simulink model "ArrayMaker"  (R2021a)
settings: Solver=FixedStepAuto  StartTime=0.0  StopTime=inf  RelTol=1e-3
model workspace (MAT data in the model file):
  Logfile_Data_Object = robotics.ros.BagSelection
  Logfile_Data_Object.FilePath = 'C:\Users\yekat\Documents\MATLAB source files\Pioneer Files\Rosbag files\November\01.11.22\Point A-B part 1.bag'
  Logfile_Data_Object.StartTime = 1663346854.77
  Logfile_Data_Object.EndTime = 1663347023.11
  Logfile_Data_Object.NumMessages = 14261
  Logfile_Data_Object.AvailableTopics = table
  Logfile_Data_Object.AvailableTopics.data{1} = [1; 1681; 1681; 1385; 1; 1; 1; 1682; 1681; 1682; 1397; 1385; 1683]
  Logfile_Data_Object.AvailableTopics.data{2} = categorical
  Logfile_Data_Object.AvailableTopics.data{2}.categoryNames = {'dynamic_reconfigure/Config'; 'dynamic_reconfigure/ConfigDescription'; 'geometry_msgs/Twist'; 'nav_msgs/Odometry'; 'rosaria/BumperState'; 'rosgraph_msgs/Log'; 'sensor_msgs/PointCloud'; 'sensor_msgs/PointCloud2'; 'std_msgs/Bool'; 'std_msgs/Float64'; 'std_msgs/Int8'; 'tf2_msgs/TFMessage'}
  Logfile_Data_Object.AvailableTopics.data{2}.codes = [11; 10; 5; 3; 9; 2; 1; 4; 7; 8; 6; 6; 12]
  Logfile_Data_Object.AvailableTopics.data{3}{1} = ''
  Logfile_Data_Object.AvailableTopics.data{3}{2} = ''
  Logfile_Data_Object.AvailableTopics.data{3}{3} = '  uint32 Seq
    |   Time Stamp
    |   char FrameId
    | logical[] FrontBumpers
    | logical[] RearBumpers
    | '
  Logfile_Data_Object.AvailableTopics.data{3}{4} = '  double X
    |   double Y
    |   double Z
    | geometry_msgs/Vector3 Angular
    |   double X
    |   double Y
    |   double Z
    | '
  Logfile_Data_Object.AvailableTopics.data{3}{5} = ''
  Logfile_Data_Object.AvailableTopics.data{3}{6} = '  char Name
    |   char Type
    |   dynamic_reconfigure/ParamDescription[] Parameters
    |     char Name
    |     char Type
    |     uint32 Level
    |     char Description
    |     char EditMethod
    |   int32 Parent
    |   int32 Id
    | dynamic_reconfigure/Config Max
    |   dynamic_reconfigure/BoolParameter[] Bools
    |     char Name
    |     logical Value
    |   dynamic_reconfigure/IntParameter[] Ints
    |     char Name
    |     int32 Value
    |   dynamic_reconfigure/StrParameter[] Strs
    |     char Name
    |     char Value
    |   dynamic_reconfigure/DoubleParameter[] Doubles
    |     char Name
    |     double Value
    |   dynamic_reconfigure/GroupState[] Groups
    |     char Name
    |     logical State
    |     int32 Id
    |     int32 Parent
    | dynamic_reconfigure/Config Min
    |   dynamic_reconfigure/BoolParameter[] Bools
    |     char Name
    |     logical Value
    |   dynamic_reconfigure/IntParameter[] Ints
    |     char Name
    |     int32 Value
    |   dynamic_reconfigure/StrParameter[] Strs
    |     char Name
    |     char Value
    |   dynamic_reconfigure/DoubleParameter[] Doubles
    |     char Name
    |     double Value
    |   dynamic_reconfigure/GroupState[] Groups
    |     char Name
    |     logical State
    |     int32 Id
    |     int32 Parent
    | dynamic_reconfigure/Config Dflt
    |   dynamic_reconfigure/BoolParameter[] Bools
    |     char Name
    |     logical Value
    |   dynamic_reconfigure/IntParameter[] Ints
    |     char Name
    |     int32 Value
    |   dynamic_reconfigure/StrParameter[] Strs
    |     char Name
    |     char Value
    |   dynamic_reconfigure/DoubleParameter[] Doubles
    |     char Name
    |     double Value
    |   dynamic_reconfigure/GroupState[] Groups
    |     char Name
    |     logical State
    |     int32 Id
    |     int32 Parent
    | '
  Logfile_Data_Object.AvailableTopics.data{3}{7} = '  char Name
    |   logical Value
    | dynamic_reconfigure/IntParameter[] Ints
    |   char Name
    |   int32 Value
    | dynamic_reconfigure/StrParameter[] Strs
    |   char Name
    |   char Value
    | dynamic_reconfigure/DoubleParameter[] Doubles
    |   char Name
    |   double Value
    | dynamic_reconfigure/GroupState[] Groups
    |   char Name
    |   logical State
    |   int32 Id
    |   int32 Parent
    | '
  Logfile_Data_Object.AvailableTopics.data{3}{8} = '  uint32 Seq
    |   Time Stamp
    |   char FrameId
    | char ChildFrameId
    | geometry_msgs/PoseWithCovariance Pose
    |   geometry_msgs/Pose Pose
    |     geometry_msgs/Point Position
    |       double X
    |       double Y
    |       double Z
    |     geometry_msgs/Quaternion Orientation
    |       double X
    |       double Y
    |       double Z
    |       double W
    |   double[36] Covariance
    | geometry_msgs/TwistWithCovariance Twist
    |   geometry_msgs/Twist Twist
    |     geometry_msgs/Vector3 Linear
    |       double X
    |       double Y
    |       double Z
    |     geometry_msgs/Vector3 Angular
    |       double X
    |       double Y
    |       double Z
    |   double[36] Covariance
    | '
  Logfile_Data_Object.AvailableTopics.data{3}{9} = '  uint32 Seq
    |   Time Stamp
    |   char FrameId
    | geometry_msgs/Point32[] Points
    |   single X
    |   single Y
    |   single Z
    | sensor_msgs/ChannelFloat32[] Channels
    |   char Name
    |   single[] Values
    | '
  Logfile_Data_Object.AvailableTopics.data{3}{10} = '  uint32 Seq
    |   Time Stamp
    |   char FrameId
    | uint32 Height
    | uint32 Width
    | sensor_msgs/PointField[] Fields
    |   uint8 INT8
    |   uint8 UINT8
    |   uint8 INT16
    |   uint8 UINT16
    |   uint8 INT32
    |   uint8 UINT32
    |   uint8 FLOAT32
    |   uint8 FLOAT64
    |   char Name
    |   uint32 Offset
    |   uint8 Datatype
    |   uint32 Count
    | logical IsBigendian
    | uint32 PointStep
    | uint32 RowStep
    | uint8[] Data
    | logical IsDense
    | '
  Logfile_Data_Object.AvailableTopics.data{3}{11} = 'int8 INFO
    | int8 WARN
    | int8 ERROR
    | int8 FATAL
    | std_msgs/Header Header
    |   uint32 Seq
    |   Time Stamp
    |   char FrameId
    | int8 Level
    | char Name
    | char Msg
    | char File
    | char Function
    | uint32 Line
    | char[] Topics
    | '
  Logfile_Data_Object.AvailableTopics.data{3}{12} = 'int8 INFO
    | int8 WARN
    | int8 ERROR
    | int8 FATAL
    | std_msgs/Header Header
    |   uint32 Seq
    |   Time Stamp
    |   char FrameId
    | int8 Level
    | char Name
    | char Msg
    | char File
    | char Function
    | uint32 Line
    | char[] Topics
    | '
  Logfile_Data_Object.AvailableTopics.data{3}{13} = '  std_msgs/Header Header
    |     uint32 Seq
    |     Time Stamp
    |     char FrameId
    |   char ChildFrameId
    |   geometry_msgs/Transform Transform
    |     geometry_msgs/Vector3 Translation
    |       double X
    |       double Y
    |       double Z
    |     geometry_msgs/Quaternion Rotation
    |       double X
    |       double Y
    |       double Z
    |       double W
    | '
  Logfile_Data_Object.AvailableTopics.ndims = 2
  Logfile_Data_Object.AvailableTopics.nrows = 13
  Logfile_Data_Object.AvailableTopics.rownames = {'/RosAria/battery_recharge_state'; '/RosAria/battery_voltage'; '/RosAria/bumper_state'; '/RosAria/cmd_vel'; '/RosAria/motors_state'; '/RosAria/parameter_descriptions'; '/RosAria/parameter_updates'; '/RosAria/pose'; '/RosAria/sonar'; '/RosAria/sonar_pointcloud2'; '/rosout'; '/rosout_agg'; '/tf'}
  Logfile_Data_Object.AvailableTopics.nvars = 3
  Logfile_Data_Object.AvailableTopics.varnames = {'NumMessages', 'MessageType', 'MessageDefinition'}
  Logfile_Data_Object.AvailableTopics.props.useVariableNamesOriginal = 0
  Logfile_Data_Object.AvailableTopics.props.useDimensionNamesOriginal = 0
  Logfile_Data_Object.AvailableTopics.props.CustomProps = struct()
  Logfile_Data_Object.AvailableTopics.props.VariableCustomProps = struct()
  Logfile_Data_Object.AvailableTopics.props.versionSavedFrom = 4
  Logfile_Data_Object.AvailableTopics.props.minCompatibleVersion = 1
  Logfile_Data_Object.AvailableTopics.props.incompatibilityMsg = ''
  Logfile_Data_Object.AvailableTopics.props.VersionSavedFrom = 4
  Logfile_Data_Object.AvailableTopics.props.Description = ''
  Logfile_Data_Object.AvailableTopics.props.VariableNamesOriginal = {}
  Logfile_Data_Object.AvailableTopics.props.DimensionNames = {'Row', 'Variables'}
  Logfile_Data_Object.AvailableTopics.props.DimensionNamesOriginal = {}
  Logfile_Data_Object.AvailableTopics.props.UserData = []
  Logfile_Data_Object.AvailableTopics.props.VariableDescriptions = {}
  Logfile_Data_Object.AvailableTopics.props.VariableUnits = {}
  Logfile_Data_Object.AvailableTopics.props.VariableContinuity = {}
  Logfile_Data_Object.AvailableFrames = {'base_link'; 'odom'}
  Logfile_Data_Object.MessageList = table
  Logfile_Data_Object.MessageList.data{1} = [1663346854.77 1663346854.77 1663346854.77 1663346854.77 1663346854.77 1663346854.77 1663346854.77 1663346854.77 1663346854.77 1663346854.77 1663346854.78 1663346854.78 ... (14261 elements, 14261x1)]
  Logfile_Data_Object.MessageList.data{2} = categorical
  Logfile_Data_Object.MessageList.data{2}.categoryNames = {'/RosAria/battery_recharge_state'; '/RosAria/battery_voltage'; '/RosAria/bumper_state'; '/RosAria/cmd_vel'; '/RosAria/motors_state'; '/RosAria/parameter_descriptions'; '/RosAria/parameter_updates'; '/RosAria/pose'; '/RosAria/sonar'; '/RosAria/sonar_pointcloud2'; '/rosout'; '/rosout_agg'; '/tf'}
  Logfile_Data_Object.MessageList.data{2}.codes = [11 11 11 11 11 11 11 11 11 11 6 5 ... (14261 elements, 14261x1)]
  Logfile_Data_Object.MessageList.data{3} = categorical
  Logfile_Data_Object.MessageList.data{3}.categoryNames = {'std_msgs/Int8'; 'std_msgs/Float64'; 'rosaria/BumperState'; 'geometry_msgs/Twist'; 'std_msgs/Bool'; 'dynamic_reconfigure/ConfigDescription'; 'dynamic_reconfigure/Config'; 'nav_msgs/Odometry'; 'sensor_msgs/PointCloud'; 'sensor_msgs/PointCloud2'; 'rosgraph_msgs/Log'; 'tf2_msgs/TFMessage'}
  Logfile_Data_Object.MessageList.data{3}.codes = [11 11 11 11 11 11 11 11 11 11 6 5 ... (14261 elements, 14261x1)]
  Logfile_Data_Object.MessageList.data{4} = [5486 5746 6002 6281 6566 6840 7104 7381 7665 7932 9864 11694 ... (14261 elements, 14261x1)]
  Logfile_Data_Object.MessageList.ndims = 2
  Logfile_Data_Object.MessageList.nrows = 14261
  Logfile_Data_Object.MessageList.nvars = 4
  Logfile_Data_Object.MessageList.varnames = {'Time', 'Topic', 'MessageType', 'FileOffset'}
  Logfile_Data_Object.MessageList.props.useVariableNamesOriginal = 0
  Logfile_Data_Object.MessageList.props.useDimensionNamesOriginal = 0
  Logfile_Data_Object.MessageList.props.CustomProps = struct()
  Logfile_Data_Object.MessageList.props.VariableCustomProps = struct()
  Logfile_Data_Object.MessageList.props.versionSavedFrom = 4
  Logfile_Data_Object.MessageList.props.minCompatibleVersion = 1
  Logfile_Data_Object.MessageList.props.incompatibilityMsg = ''
  Logfile_Data_Object.MessageList.props.VersionSavedFrom = 4
  Logfile_Data_Object.MessageList.props.Description = ''
  Logfile_Data_Object.MessageList.props.VariableNamesOriginal = {}
  Logfile_Data_Object.MessageList.props.DimensionNames = {'Row', 'Variables'}
  Logfile_Data_Object.MessageList.props.DimensionNamesOriginal = {}
  Logfile_Data_Object.MessageList.props.UserData = []
  Logfile_Data_Object.MessageList.props.VariableDescriptions = {}
  Logfile_Data_Object.MessageList.props.VariableUnits = {}
  Logfile_Data_Object.MessageList.props.VariableContinuity = {}
  Logfile_Data_Object.TopicTypeMap = containers.Map
  Logfile_Data_Object.TopicTypeMap.serialization.keys = {'/RosAria/battery_recharge_state', '/RosAria/battery_voltage', '/RosAria/bumper_state', '/RosAria/cmd_vel', '/RosAria/motors_state', '/RosAria/parameter_descriptions', '/RosAria/parameter_updates', '/RosAria/pose', '/RosAria/sonar', '/RosAria/sonar_pointcloud2', '/rosout', '/rosout_agg', '/tf'}
  Logfile_Data_Object.TopicTypeMap.serialization.values = {'std_msgs/Int8', 'std_msgs/Float64', 'rosaria/BumperState', 'geometry_msgs/Twist', 'std_msgs/Bool', 'dynamic_reconfigure/ConfigDescription', 'dynamic_reconfigure/Config', 'nav_msgs/Odometry', 'sensor_msgs/PointCloud', 'sensor_msgs/PointCloud2', 'rosgraph_msgs/Log', 'rosgraph_msgs/Log', 'tf2_msgs/TFMessage'}
  Logfile_Data_Object.TopicTypeMap.serialization.uniformity = 1
  Logfile_Data_Object.TopicTypeMap.serialization.keyType = 'char'
  Logfile_Data_Object.TopicTypeMap.serialization.valueType = 'char'
  Logfile_Data_Object.TopicDefinitionMap = containers.Map
  Logfile_Data_Object.TopicDefinitionMap.serialization.keys = {'/RosAria/battery_recharge_state', '/RosAria/battery_voltage', '/RosAria/bumper_state', '/RosAria/cmd_vel', '/RosAria/motors_state', '/RosAria/parameter_descriptions', '/RosAria/parameter_updates', '/RosAria/pose', '/RosAria/sonar', '/RosAria/sonar_pointcloud2', '/rosout', '/rosout_agg', '/tf'}
  Logfile_Data_Object.TopicDefinitionMap.serialization.values{1} = ''
  Logfile_Data_Object.TopicDefinitionMap.serialization.values{2} = ''
  Logfile_Data_Object.TopicDefinitionMap.serialization.values{3} = '  uint32 Seq
    |   Time Stamp
    |   char FrameId
    | logical[] FrontBumpers
    | logical[] RearBumpers
    | '
  Logfile_Data_Object.TopicDefinitionMap.serialization.values{4} = '  double X
    |   double Y
    |   double Z
    | geometry_msgs/Vector3 Angular
    |   double X
    |   double Y
    |   double Z
    | '
  Logfile_Data_Object.TopicDefinitionMap.serialization.values{5} = ''
  Logfile_Data_Object.TopicDefinitionMap.serialization.values{6} = '  char Name
    |   char Type
    |   dynamic_reconfigure/ParamDescription[] Parameters
    |     char Name
    |     char Type
    |     uint32 Level
    |     char Description
    |     char EditMethod
    |   int32 Parent
    |   int32 Id
    | dynamic_reconfigure/Config Max
    |   dynamic_reconfigure/BoolParameter[] Bools
    |     char Name
    |     logical Value
    |   dynamic_reconfigure/IntParameter[] Ints
    |     char Name
    |     int32 Value
    |   dynamic_reconfigure/StrParameter[] Strs
    |     char Name
    |     char Value
    |   dynamic_reconfigure/DoubleParameter[] Doubles
    |     char Name
    |     double Value
    |   dynamic_reconfigure/GroupState[] Groups
    |     char Name
    |     logical State
    |     int32 Id
    |     int32 Parent
    | dynamic_reconfigure/Config Min
    |   dynamic_reconfigure/BoolParameter[] Bools
    |     char Name
    |     logical Value
    |   dynamic_reconfigure/IntParameter[] Ints
    |     char Name
    |     int32 Value
    |   dynamic_reconfigure/StrParameter[] Strs
    |     char Name
    |     char Value
    |   dynamic_reconfigure/DoubleParameter[] Doubles
    |     char Name
    |     double Value
    |   dynamic_reconfigure/GroupState[] Groups
    |     char Name
    |     logical State
    |     int32 Id
    |     int32 Parent
    | dynamic_reconfigure/Config Dflt
    |   dynamic_reconfigure/BoolParameter[] Bools
    |     char Name
    |     logical Value
    |   dynamic_reconfigure/IntParameter[] Ints
    |     char Name
    |     int32 Value
    |   dynamic_reconfigure/StrParameter[] Strs
    |     char Name
    |     char Value
    |   dynamic_reconfigure/DoubleParameter[] Doubles
    |     char Name
    |     double Value
    |   dynamic_reconfigure/GroupState[] Groups
    |     char Name
    |     logical State
    |     int32 Id
    |     int32 Parent
    | '
  Logfile_Data_Object.TopicDefinitionMap.serialization.values{7} = '  char Name
    |   logical Value
    | dynamic_reconfigure/IntParameter[] Ints
    |   char Name
    |   int32 Value
    | dynamic_reconfigure/StrParameter[] Strs
    |   char Name
    |   char Value
    | dynamic_reconfigure/DoubleParameter[] Doubles
    |   char Name
    |   double Value
    | dynamic_reconfigure/GroupState[] Groups
    |   char Name
    |   logical State
    |   int32 Id
    |   int32 Parent
    | '
  Logfile_Data_Object.TopicDefinitionMap.serialization.values{8} = '  uint32 Seq
    |   Time Stamp
    |   char FrameId
    | char ChildFrameId
    | geometry_msgs/PoseWithCovariance Pose
    |   geometry_msgs/Pose Pose
    |     geometry_msgs/Point Position
    |       double X
    |       double Y
    |       double Z
    |     geometry_msgs/Quaternion Orientation
    |       double X
    |       double Y
    |       double Z
    |       double W
    |   double[36] Covariance
    | geometry_msgs/TwistWithCovariance Twist
    |   geometry_msgs/Twist Twist
    |     geometry_msgs/Vector3 Linear
    |       double X
    |       double Y
    |       double Z
    |     geometry_msgs/Vector3 Angular
    |       double X
    |       double Y
    |       double Z
    |   double[36] Covariance
    | '
  Logfile_Data_Object.TopicDefinitionMap.serialization.values{9} = '  uint32 Seq
    |   Time Stamp
    |   char FrameId
    | geometry_msgs/Point32[] Points
    |   single X
    |   single Y
    |   single Z
    | sensor_msgs/ChannelFloat32[] Channels
    |   char Name
    |   single[] Values
    | '
  Logfile_Data_Object.TopicDefinitionMap.serialization.values{10} = '  uint32 Seq
    |   Time Stamp
    |   char FrameId
    | uint32 Height
    | uint32 Width
    | sensor_msgs/PointField[] Fields
    |   uint8 INT8
    |   uint8 UINT8
    |   uint8 INT16
    |   uint8 UINT16
    |   uint8 INT32
    |   uint8 UINT32
    |   uint8 FLOAT32
    |   uint8 FLOAT64
    |   char Name
    |   uint32 Offset
    |   uint8 Datatype
    |   uint32 Count
    | logical IsBigendian
    | uint32 PointStep
    | uint32 RowStep
    | uint8[] Data
    | logical IsDense
    | '
  Logfile_Data_Object.TopicDefinitionMap.serialization.values{11} = 'int8 INFO
    | int8 WARN
    | int8 ERROR
    | int8 FATAL
    | std_msgs/Header Header
    |   uint32 Seq
    |   Time Stamp
    |   char FrameId
    | int8 Level
    | char Name
    | char Msg
    | char File
    | char Function
    | uint32 Line
    | char[] Topics
    | '
  Logfile_Data_Object.TopicDefinitionMap.serialization.values{12} = 'int8 INFO
    | int8 WARN
    | int8 ERROR
    | int8 FATAL
    | std_msgs/Header Header
    |   uint32 Seq
    |   Time Stamp
    |   char FrameId
    | int8 Level
    | char Name
    | char Msg
    | char File
    | char Function
    | uint32 Line
    | char[] Topics
    | '
  Logfile_Data_Object.TopicDefinitionMap.serialization.values{13} = '  std_msgs/Header Header
    |     uint32 Seq
    |     Time Stamp
    |     char FrameId
    |   char ChildFrameId
    |   geometry_msgs/Transform Transform
    |     geometry_msgs/Vector3 Translation
    |       double X
    |       double Y
    |       double Z
    |     geometry_msgs/Quaternion Rotation
    |       double X
    |       double Y
    |       double Z
    |       double W
    | '
  Logfile_Data_Object.TopicDefinitionMap.serialization.uniformity = 1
  Logfile_Data_Object.TopicDefinitionMap.serialization.keyType = 'char'
  Logfile_Data_Object.TopicDefinitionMap.serialization.valueType = 'char'
  Logfile_Data_Object.messageTypeMap = containers.Map
  Logfile_Data_Object.messageTypeMap.serialization.keys = {}
  Logfile_Data_Object.messageTypeMap.serialization.values = {}
  Logfile_Data_Object.messageTypeMap.serialization.uniformity = 0
  Logfile_Data_Object.messageTypeMap.serialization.keyType = 'char'
  Logfile_Data_Object.messageTypeMap.serialization.valueType = 'any'
  Logfile_Data_Object.Parser = robotics.ros.internal.tf.TransformationTreeParser
  Logfile_Data_Object.Parser.UseObjectMsg = 1
  Logfile_Path = 'C:\Users\yekat\Documents\MATLAB source files\Pioneer Files\Rosbag files\November\01.11.22\Point A-B part 1.bag'
  Logfile_Playback_Duration = nan
  Logfile_Playback_Offset = nan
libraries: robotlib x2
settings Model: Creator=yekat  LastModifiedBy=yekat
settings OptimizationCC: EnhancedBackFolding=on  PassReuseOutputArgsAs=Individual arguments  ZeroExternalMemoryAtStartup=off  ZeroInternalMemoryAtStartup=off  MaxStackSize=64  OptimizeBlockOrder=speed  DifferentSizesBufferReuse=on  OptimizationCustomize=off  EfficientTunableParamExpr=on
settings DebuggingCC: ParameterTunabilityLossMsg=error
settings HardwareCC: ProdBitPerPointer=32  ProdBitPerSizeT=32  ProdBitPerPtrDiffT=32  ProdLargestAtomicFloat=None  ProdIntDivRoundTo=Undefined  ProdEndianess=Unspecified  ProdWordSize=32  ProdHWDeviceType=Generic->Unspecified (assume 32-bit Generic)
settings SFSimCC: MATLABDynamicMemAlloc=off
settings RTWCC: SystemTargetFile=ert.tlc  HardwareBoard=Robot Operating System (ROS)  TLCOptions="-aInlineSetEventsForThisBaseRateFcn=TLC_FALSE -aSuppressMultiTaskScheduler=TLC_FALSE  -aRateBasedStepFcn=0"  TemplateMakefile=ert_default_tmf  Toolchain=Catkin  TargetLang=C++
settings CodeAppCC: ForceParamTrailComments=on  IgnoreCustomStorageClasses=off  OperatorAnnotations=on  SimulinkDataObjDesc=on  SFDataObjDesc=on  InsertBlockDesc=on

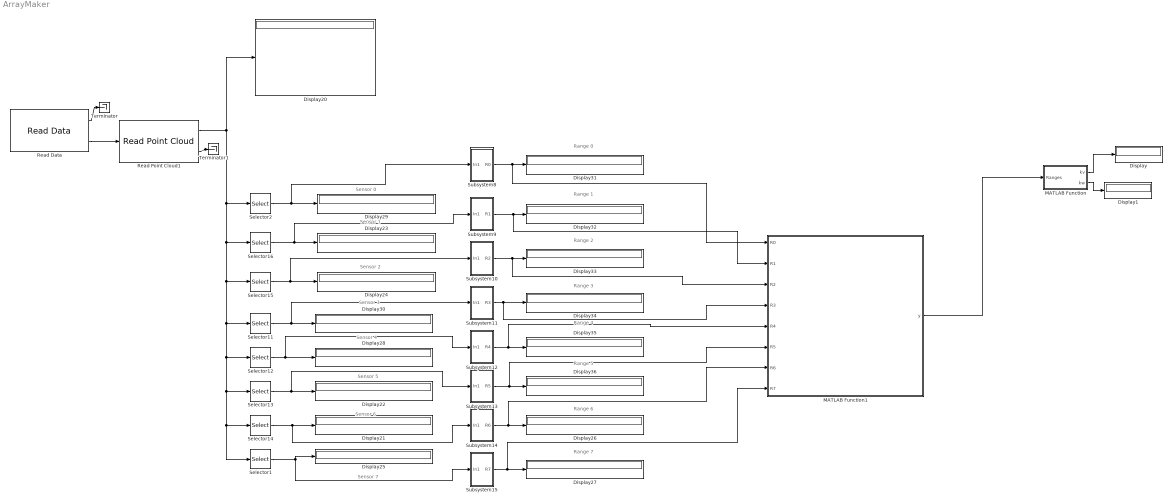
== system ArrayMaker ==
  note: Sensor 6
  note: Range 4
  note: Sensor 0
  note: Sensor 5
  note: Sensor 7
  note: Range 2
  note: Range 1
  note: Range 0
  note: Sensor 1
  note: Range 7
  note: Range 5
  note: Range 6
  note: Sensor 3
  note: Sensor 4
  note: Range 3
  note: Sensor 2
  Display{,1,20..36} (19 alike) : Display
  MATLAB Function : MATLAB Function  TreatAsAtomicUnit=on
  MATLAB Function1 : MATLAB Function  TreatAsAtomicUnit=on
  Read Data : robotlib/Read Data  topic=/RosAria/sonar_pointcloud2  sampleTime=-1  logfileType=rosbag  modelName=ArrayMaker  msgType=sensor_msgs/PointCloud2
      settings: SourceProductBaseCode=RR
  Read Point Cloud1 : robotlib/Read Point Cloud  MaximumPointCloudSize=[8, 1]  PreserveStructure=off  ShowRGBOutput=off  ShowIntensityOutput=off  ShowErrorCodeOutput=on  VariableSizeOutputs=off
      settings: SourceProductBaseCode=RR
  Selector1 : Selector  NumberOfDimensions=2  InputPortWidth=6  IndexOptions=Starting index (dialog),Starting index (dialog)  Indices=8,1  OutputSizes=1,3
  Selector11 : Selector  NumberOfDimensions=2  InputPortWidth=6  IndexOptions=Starting index (dialog),Starting index (dialog)  Indices=4,1  OutputSizes=1,3
  Selector12 : Selector  NumberOfDimensions=2  InputPortWidth=6  IndexOptions=Starting index (dialog),Starting index (dialog)  Indices=5,1  OutputSizes=1,3
  Selector13 : Selector  NumberOfDimensions=2  InputPortWidth=6  IndexOptions=Starting index (dialog),Starting index (dialog)  Indices=6,1  OutputSizes=1,3
  Selector14 : Selector  NumberOfDimensions=2  InputPortWidth=6  IndexOptions=Starting index (dialog),Starting index (dialog)  Indices=7,1  OutputSizes=1,3
  Selector15 : Selector  NumberOfDimensions=2  InputPortWidth=6  IndexOptions=Starting index (dialog),Starting index (dialog)  Indices=3,1  OutputSizes=1,3
  Selector16 : Selector  NumberOfDimensions=2  InputPortWidth=6  IndexOptions=Starting index (dialog),Starting index (dialog)  Indices=2,1  OutputSizes=1,3
  Selector2 : Selector  NumberOfDimensions=2  InputPortWidth=6  IndexOptions=Starting index (dialog),Starting index (dialog)  Indices=1,1  OutputSizes=1,3
  Subsystem10 : Subsystem
  Subsystem11 : Subsystem
  Subsystem12 : Subsystem
  Subsystem13 : Subsystem
  Subsystem14 : Subsystem
  Subsystem15 : Subsystem
  Subsystem8 : Subsystem
  Subsystem9 : Subsystem
  Terminator : Terminator
  Terminator1 : Terminator
  wires:
  MATLAB Function/2(kw) -> Display1/1
  MATLAB Function/1(kv) -> Display/1
  Read Data/2 -> Read Point Cloud1/1
  Read Point Cloud1/1 -> Selector1/1, Selector14/1, Selector13/1, Selector12/1, Selector11/1, Selector15/1, Selector16/1, Selector2/1, Display20/1
  Subsystem8/1(R0) -> MATLAB Function1/1(R0), Display31/1
  Selector16/1 -> Subsystem9/1(In1), Display23/1
  Selector12/1 -> Subsystem12/1(In1), Display28/1
  Subsystem11/1(R3) -> MATLAB Function1/4(R3), Display34/1
  Selector1/1 -> Subsystem15/1(In1), Display25/1
  Selector14/1 -> Subsystem14/1(In1), Display21/1
  Subsystem14/1(R6) -> MATLAB Function1/7(R6), Display26/1
  Subsystem10/1(R2) -> MATLAB Function1/3(R2), Display33/1
  Selector2/1 -> Subsystem8/1(In1), Display29/1
  Selector11/1 -> Subsystem11/1(In1), Display30/1
  Subsystem9/1(R1) -> MATLAB Function1/2(R1), Display32/1
  Subsystem13/1(R5) -> MATLAB Function1/6(R5), Display36/1
  Selector13/1 -> Subsystem13/1(In1), Display22/1
  Subsystem12/1(R4) -> MATLAB Function1/5(R4), Display35/1
  Selector15/1 -> Subsystem10/1(In1), Display24/1
  Subsystem15/1(R7) -> MATLAB Function1/8(R7), Display27/1
  MATLAB Function1/1(y) -> MATLAB Function/1(Ranges)
  Read Data/1 -> Terminator/1
  Read Point Cloud1/2 -> Terminator1/1

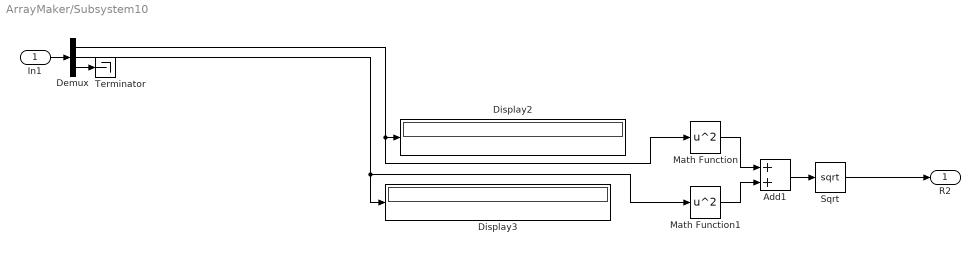
== system ArrayMaker/Subsystem10 ==
  In1 : Inport
  Add1 : Sum
  Demux : Demux  Outputs=3
  Display2 : Display
  Display3 : Display
  Math Function : Math  Operator=square  SaturateOnIntegerOverflow=on
  Math Function1 : Math  Operator=square  SaturateOnIntegerOverflow=on
  Sqrt : Sqrt  SaturateOnIntegerOverflow=on
  Terminator : Terminator
  R2 : Outport
  wires:
  Math Function1/1 -> Add1/2
  Demux/1 -> Math Function/1, Display2/1
  In1/1 -> Demux/1
  Math Function/1 -> Add1/1
  Demux/2 -> Display3/1, Math Function1/1
  Sqrt/1 -> R2/1
  Add1/1 -> Sqrt/1
  Demux/3 -> Terminator/1

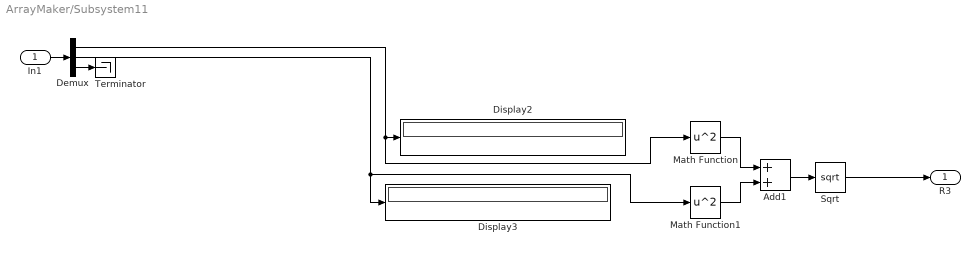
== system ArrayMaker/Subsystem11 ==
  In1 : Inport
  Add1 : Sum
  Demux : Demux  Outputs=3
  Display2 : Display
  Display3 : Display
  Math Function : Math  Operator=square  SaturateOnIntegerOverflow=on
  Math Function1 : Math  Operator=square  SaturateOnIntegerOverflow=on
  Sqrt : Sqrt  SaturateOnIntegerOverflow=on
  Terminator : Terminator
  R3 : Outport
  wires:
  Math Function1/1 -> Add1/2
  Demux/1 -> Math Function/1, Display2/1
  In1/1 -> Demux/1
  Math Function/1 -> Add1/1
  Demux/2 -> Display3/1, Math Function1/1
  Sqrt/1 -> R3/1
  Add1/1 -> Sqrt/1
  Demux/3 -> Terminator/1

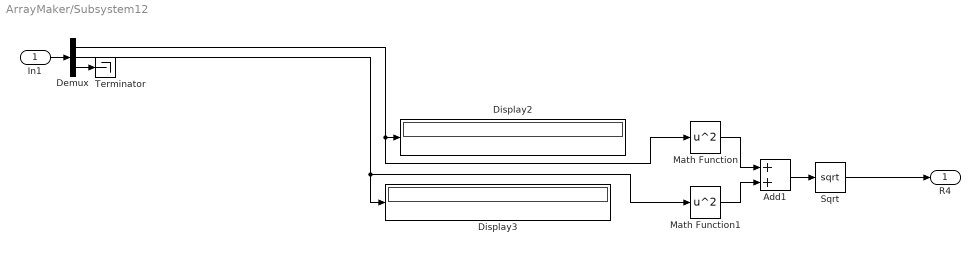
== system ArrayMaker/Subsystem12 ==
  In1 : Inport
  Add1 : Sum
  Demux : Demux  Outputs=3
  Display2 : Display
  Display3 : Display
  Math Function : Math  Operator=square  SaturateOnIntegerOverflow=on
  Math Function1 : Math  Operator=square  SaturateOnIntegerOverflow=on
  Sqrt : Sqrt  SaturateOnIntegerOverflow=on
  Terminator : Terminator
  R4 : Outport
  wires:
  Math Function1/1 -> Add1/2
  Demux/1 -> Math Function/1, Display2/1
  In1/1 -> Demux/1
  Math Function/1 -> Add1/1
  Demux/2 -> Display3/1, Math Function1/1
  Sqrt/1 -> R4/1
  Add1/1 -> Sqrt/1
  Demux/3 -> Terminator/1

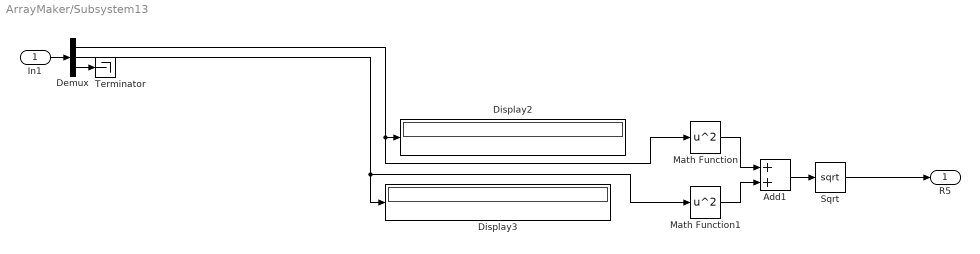
== system ArrayMaker/Subsystem13 ==
  In1 : Inport
  Add1 : Sum
  Demux : Demux  Outputs=3
  Display2 : Display
  Display3 : Display
  Math Function : Math  Operator=square  SaturateOnIntegerOverflow=on
  Math Function1 : Math  Operator=square  SaturateOnIntegerOverflow=on
  Sqrt : Sqrt  SaturateOnIntegerOverflow=on
  Terminator : Terminator
  R5 : Outport
  wires:
  Math Function1/1 -> Add1/2
  Demux/1 -> Math Function/1, Display2/1
  In1/1 -> Demux/1
  Math Function/1 -> Add1/1
  Demux/2 -> Display3/1, Math Function1/1
  Sqrt/1 -> R5/1
  Add1/1 -> Sqrt/1
  Demux/3 -> Terminator/1

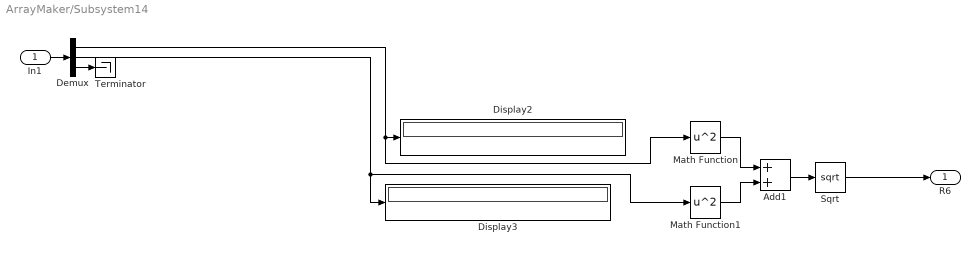
== system ArrayMaker/Subsystem14 ==
  In1 : Inport
  Add1 : Sum
  Demux : Demux  Outputs=3
  Display2 : Display
  Display3 : Display
  Math Function : Math  Operator=square  SaturateOnIntegerOverflow=on
  Math Function1 : Math  Operator=square  SaturateOnIntegerOverflow=on
  Sqrt : Sqrt  SaturateOnIntegerOverflow=on
  Terminator : Terminator
  R6 : Outport
  wires:
  Math Function1/1 -> Add1/2
  Demux/1 -> Math Function/1, Display2/1
  In1/1 -> Demux/1
  Math Function/1 -> Add1/1
  Demux/2 -> Display3/1, Math Function1/1
  Sqrt/1 -> R6/1
  Add1/1 -> Sqrt/1
  Demux/3 -> Terminator/1

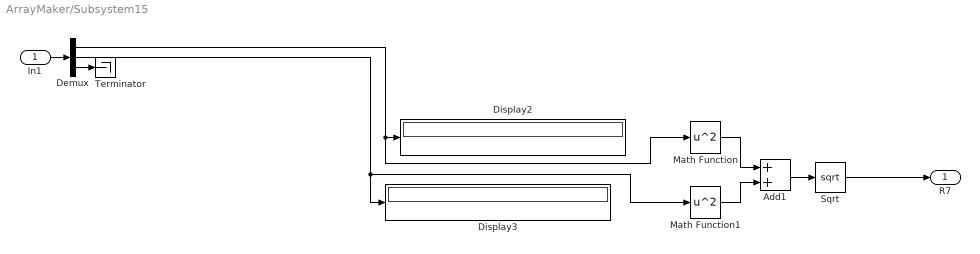
== system ArrayMaker/Subsystem15 ==
  In1 : Inport
  Add1 : Sum
  Demux : Demux  Outputs=3
  Display2 : Display
  Display3 : Display
  Math Function : Math  Operator=square  SaturateOnIntegerOverflow=on
  Math Function1 : Math  Operator=square  SaturateOnIntegerOverflow=on
  Sqrt : Sqrt  SaturateOnIntegerOverflow=on
  Terminator : Terminator
  R7 : Outport
  wires:
  Math Function1/1 -> Add1/2
  Demux/1 -> Math Function/1, Display2/1
  In1/1 -> Demux/1
  Math Function/1 -> Add1/1
  Demux/2 -> Display3/1, Math Function1/1
  Sqrt/1 -> R7/1
  Add1/1 -> Sqrt/1
  Demux/3 -> Terminator/1

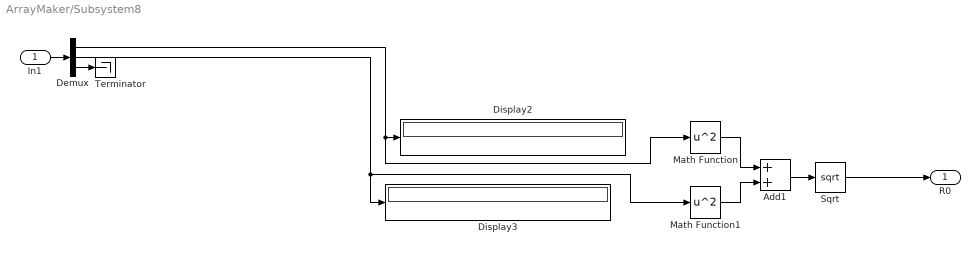
== system ArrayMaker/Subsystem8 ==
  In1 : Inport
  Add1 : Sum
  Demux : Demux  Outputs=3
  Display2 : Display
  Display3 : Display
  Math Function : Math  Operator=square  SaturateOnIntegerOverflow=on
  Math Function1 : Math  Operator=square  SaturateOnIntegerOverflow=on
  Sqrt : Sqrt  SaturateOnIntegerOverflow=on
  Terminator : Terminator
  R0 : Outport
  wires:
  Math Function1/1 -> Add1/2
  Demux/1 -> Math Function/1, Display2/1
  In1/1 -> Demux/1
  Math Function/1 -> Add1/1
  Demux/2 -> Display3/1, Math Function1/1
  Sqrt/1 -> R0/1
  Add1/1 -> Sqrt/1
  Demux/3 -> Terminator/1

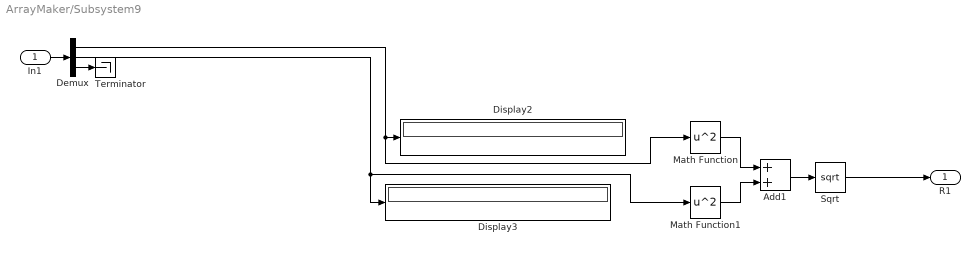
== system ArrayMaker/Subsystem9 ==
  In1 : Inport
  Add1 : Sum
  Demux : Demux  Outputs=3
  Display2 : Display
  Display3 : Display
  Math Function : Math  Operator=square  SaturateOnIntegerOverflow=on
  Math Function1 : Math  Operator=square  SaturateOnIntegerOverflow=on
  Sqrt : Sqrt  SaturateOnIntegerOverflow=on
  Terminator : Terminator
  R1 : Outport
  wires:
  Math Function1/1 -> Add1/2
  Demux/1 -> Math Function/1, Display2/1
  In1/1 -> Demux/1
  Math Function/1 -> Add1/1
  Demux/2 -> Display3/1, Math Function1/1
  Sqrt/1 -> R1/1
  Add1/1 -> Sqrt/1
  Demux/3 -> Terminator/1

== matlab function ArrayMaker/MATLAB Function1 ==
  data: R0 input; R1 input; R2 input; R3 input; R4 input; R5 input; R6 input; y output; R7 input
function y = array(R0,R1,R2,R3,R4,R5,R6,R7)
Ranges=[R0,R1,R2,R3,R4,R5,R6,R7]


y = Ranges;
end

== matlab function ArrayMaker/MATLAB Function ==
  data: Ranges input; kv output; kw output
function [kv,kw] = stopRobot(Ranges)
kv=nan;% for the case if the both conditions are false
kw=nan;
limit1=4;% Limit for sensors R3,R4
limit2=3.5;% Limit for sensors R2,R5
a=0;
while a<32
    k=(Ranges(5)<limit1)|| (Ranges(4)<limit1)||(Ranges(3)<limit2)|| (Ranges(6)<limit2);
        if k==false  
            kv=1;
            kw=1;
        else 
            kv=0;
            kw=0;
        
        end
         a=a+1;
end

end
